simulink model "AFC_Online3"  (R2021a)
settings: Solver=VariableStepAuto  StartTime=0.0  StopTime=40.0  RelTol=1e-3
libraries: slstlib x1
settings Model: Creator=Ennio  LastModifiedBy=Ennio
settings DataIOCC: ExternalInput=[t__, u__]  SaveFormat=StructureWithTime

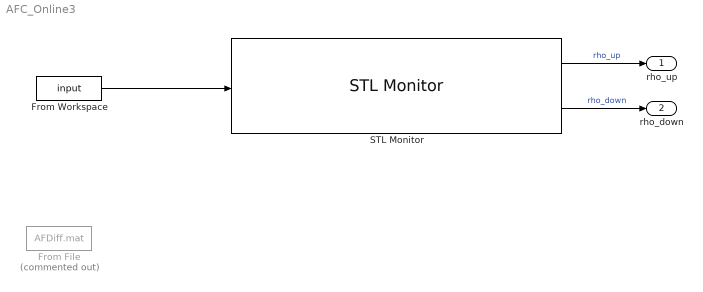
== system AFC_Online3 ==
  From Workspace : FromWorkspace  VariableName=input
  From File : FromFile  Commented=on  FileName=AFDiff.mat  SampleTime=0
  STL Monitor : slstlib/STL Monitor  SignalNames='x1,x2'  STLString='alw_[10, 30] ((x1[t] > 0.05) => (ev_[0, 1] (x1[t] < 0.05)))'  MaxRob=100  RefreshRate=0.1  rob_low_lim=inf  rob_up_lim=-inf  rob_diff_lim=-inf
      settings: SourceProductName=Breach Library
  rho_up : Outport  SignalName=rho_up
  rho_down : Outport  Port=2  SignalName=rho_down
  wires:
  STL Monitor/2 -> rho_down/1  "rho_down"
  STL Monitor/1 -> rho_up/1  "rho_up"
  From Workspace/1 -> STL Monitor/1
